simulink model "QBot2_Image_Proc_Line_Following_edited"  (R2015b)
settings: Solver=ode1  StartTime=0.0  StopTime=inf  FixedStep=0.01  RelTol=1e-3
values from neighbouring files (symbols this model uses):
  x = [0 0 0 0 0 0 0 0 0 0 0 0 ... (23417 elements, 23417x1)]    [plot_data.mat]
undefined symbols (not defined in the file or in its folder): HIL, Kinect, qc_get_step_size
libraries: quarc_library x6
settings Model: SimulationMode=external  ExtModeTrigDuration=1  Creator=drmadill  LastModifiedBy=ale
settings SolverCC: PositivePriorityOrder=on
settings DataIOCC: SaveFormat=Array  SignalLoggingSaveFormat=ModelDataLogs
settings OptimizationCC: ExpressionDepthLimit=2147483647
settings DebuggingCC: UnderspecifiedInitializationDetection=Classic  MergeDetectMultiDrivingBlocksExec=none  SolverPrmCheckMsg=warning  FcnCallInpInsideContextMsg=EnableAllAsWarning  AllowSymbolicDim=on  StateNameClashWarn=warning
settings HardwareCC: ProdBitPerPointer=32  ProdLargestAtomicFloat=None  ProdIntDivRoundTo=Undefined  ProdEndianess=Unspecified  ProdWordSize=32  ProdHWDeviceType=32-bit Generic
settings RTWCC: SystemTargetFile=quarc_linux_duovero.tlc  TemplateMakefile=quarc_linux_duovero_tmf  Description=QUARC Linux DuoVero Target
settings STFCustomTargetCC: TargetLibSuffix=.a  TargetPreCompLibLocation=C:\PROGRA~3\QUARC\lib\2015b\LINUX_~1\release  SystemTargetFile=quarc_linux_duovero.tlc
settings GRTTargetCC: TargetLibSuffix=.a  TargetPreCompLibLocation=C:\PROGRA~3\QUARC\lib\2015b\LINUX_~1\release  ParMdlRefBuildCompliant=off  CompOptLevelCompliant=off  GeneratePreprocessorConditionals=Disable all  CombineOutputUpdateFcns=off  MatFileLogging=off  GRTInterface=on  UseToolchainInfoCompliant=off  ExtMode=on  ExtModeMexFile=quarc_comm  ExtModeMexArgs='-w -d /tmp -uri %u', 'tcpip://192.168.2.51:17001'
settings ConfigComp: CovModelRefEnable=Off

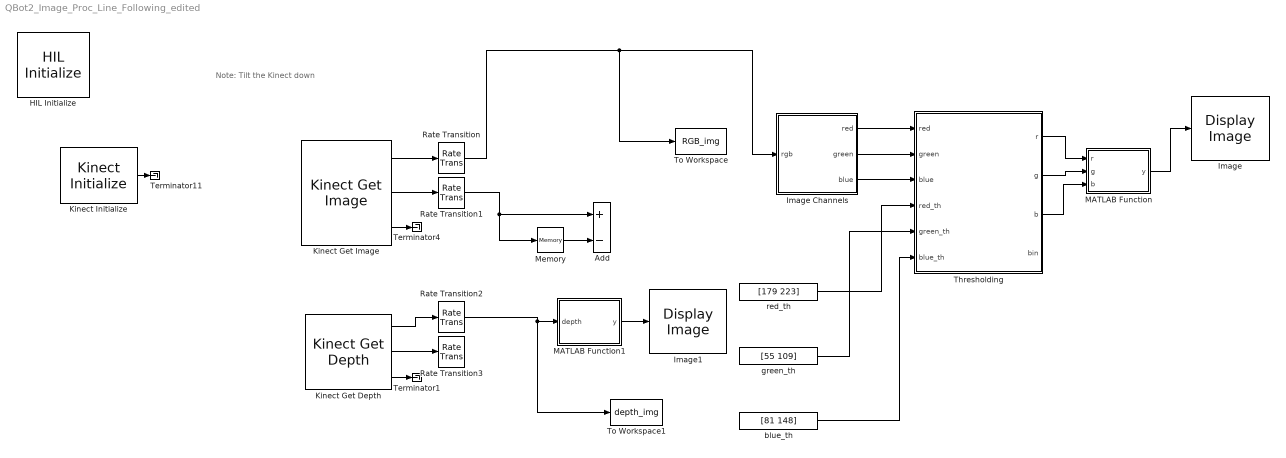
== system QBot2_Image_Proc_Line_Following_edited ==
  note: Note: Tilt the Kinect down
  Add : Sum  Inputs=+-
  HIL Initialize : quarc_library/Data Acquisition/Generic/Configuration/HIL Initialize  Priority=-99  object_name=HIL-1  board_type=qbot2  board_number=0  board_options=enc0_dir=0;enc0_filter=1;enc0_a=0;enc0_b=0;enc0_z=1;enc0_reload=0;enc1_dir=0;enc1_filter=1;enc1_a=0;enc1_b=0;enc1_z=1;enc1_reload=0;pwm0_immediate=0;pwm1_immediate=0;pwm2_immediate=0;pwm3_immediate=0;  exclusive=off  active=off  hardware_clocks=[]  clock_modes=[]  initial_clock_frequencies=[]  set_clock_params_at_start=off  set_clock_params_at_switch_in=off  set_clock_frequencies_at_start=off  set_clock_frequencies_at_switch_in=off  analog_input_channels=[0:9]  analog_input_maximums=[5 5 5 5 16.5 3.3 3.3 3.3 3.3]  analog_input_minimums=[0 0 0 0 0 0 0 0 0]  set_analog_input_params_at_start=off  set_analog_input_params_at_switch_in=off  analog_output_channels=[]  analog_output_maximums=[]  analog_output_minimums=[]  initial_analog_outputs=[]  final_analog_outputs=[]  watchdog_analog_outputs=[]  set_analog_output_params_at_start=off  set_analog_output_params_at_switch_in=off  set_analog_outputs_at_start=off  set_analog_outputs_at_switch_in=off  set_analog_outputs_at_terminate=off  set_analog_outputs_at_switch_out=off  set_analog_outputs_on_watchdog=off  digital_input_channels=[]  digital_output_channels=[]  digital_output_configuration=[]  initial_digital_outputs=[0]  final_digital_outputs=[0]  watchdog_digital_outputs=[0]  set_digital_output_params_at_start=off  set_digital_output_params_at_switch_in=off  set_digital_outputs_at_start=on  set_digital_outputs_at_switch_in=off  set_digital_outputs_at_terminate=on  set_digital_outputs_at_switch_out=off  set_digital_outputs_on_watchdog=on  encoder_channels=[0:3]  quadrature=[4]  encoder_filter_frequency=[]  initial_encoder_counts=[0]  set_encoder_params_at_start=on  set_encoder_params_at_switch_in=off  set_encoder_counts_at_start=on  set_encoder_counts_at_switch_in=off  pwm_channels=[0:3]  pwm_modes=[0]  pwm_frequency=[20e6/1024]  pwm_configuration=[0]  pwm_alignment=[0]  pwm_polarity=[1]  pwm_leading_deadband=[0]  pwm_trailing_deadband=[0]  initial_pwm_outputs=[0]  final_pwm_outputs=[0]  watchdog_pwm_outputs=[0]  set_pwm_params_at_start=on  set_pwm_params_at_switch_in=off  set_pwm_outputs_at_start=on  set_pwm_outputs_at_switch_in=off  set_pwm_outputs_at_terminate=on  set_pwm_outputs_at_switch_out=off  set_pwm_outputs_on_watchdog=on  other_output_channels=[2000:2001 14000 16000]  initial_other_outputs=[0 0 0 7]  final_other_outputs=[0 0 0 7]  watchdog_other_outputs=[]  set_other_outputs_at_start=on  set_other_outputs_at_switch_in=off  set_other_outputs_at_terminate=on  set_other_outputs_at_switch_out=off  set_other_outputs_on_watchdog=off
  Image : quarc_library/Sinks/Figures/Display Image  figure_mode=Use figure window  figure_tag=figure1  axes_tag=axes1  update_rate=1  initial_position="129  195  789  624"  initial_visibility=off  sample_time=-1  axes_only=off  orig_size=off
  Image Channels : Subsystem
  Image1 : quarc_library/Sinks/Figures/Display Image  figure_mode=Use figure window  figure_tag=figure1  axes_tag=axes1  update_rate=1  initial_position="480  173  789  624"  initial_visibility=off  sample_time=-1  axes_only=off  orig_size=off
  Kinect Get Depth : quarc_library/Multimedia/Kinect Get Depth  object_name=Kinect-1  resolution=640 x 480  sample_time=qc_get_step_size * ceil(0.033 / qc_get_step_size)  show_player=off
  Kinect Get Image : quarc_library/Multimedia/Kinect Get Image  object_name=Kinect-1  sensor_type=color  resolution=640 x 480  output_format=MATLAB RGB (HxWx3)  data_type=uint8  backlight=average brightness  flicker=none  brightness=0.2156  gain=1.0  gamma=2.2  autoexposure=on  exposure=0  contrast=1.0  sharpness=0.5  hue=0.0  saturation=1.0  autobalance=on  balance=2700  frame_interval=0  sample_time=qc_get_step_size*10
  Kinect Initialize : quarc_library/Multimedia/Kinect Initialize  object_name=Kinect-1  kinect_type=Kinect for XBox 360  identifier=0  sample_time=qc_get_step_size * 10  active=on
  MATLAB Function : MATLAB Function  TreatAsAtomicUnit=on
  MATLAB Function1 : MATLAB Function  TreatAsAtomicUnit=on
  Memory : Memory
  Rate Transition{,1..3} (4 alike) : RateTransition
  Terminator1 : Terminator
  Terminator11 : Terminator
  Terminator4 : Terminator
  Thresholding : MATLAB Function  TreatAsAtomicUnit=on
  To Workspace : ToWorkspace  VariableName=RGB_img  SampleTime=-1
      settings: MaxDataPoints=1
  To Workspace1 : ToWorkspace  VariableName=depth_img  SampleTime=-1
      settings: MaxDataPoints=1
  blue_th : Constant  Value=[81 148]
  green_th : Constant  Value=[55 109]
  red_th : Constant  Value=[179 223]
  wires:
  Kinect Get Image/1 -> Rate Transition/1
  Kinect Get Image/2 -> Rate Transition1/1
  Rate Transition1/1 -> Memory/1, Add/1
  Memory/1 -> Add/2
  Kinect Get Image/3 -> Terminator4/1
  Rate Transition/1 -> Image Channels/1(rgb), To Workspace/1
  Kinect Initialize/1 -> Terminator11/1
  Kinect Get Depth/1 -> Rate Transition2/1
  Kinect Get Depth/2 -> Rate Transition3/1
  Kinect Get Depth/3 -> Terminator1/1
  Image Channels/2(green) -> Thresholding/2(green)
  Image Channels/1(red) -> Thresholding/1(red)
  Image Channels/3(blue) -> Thresholding/3(blue)
  red_th/1 -> Thresholding/4(red_th)
  green_th/1 -> Thresholding/5(green_th)
  blue_th/1 -> Thresholding/6(blue_th)
  Thresholding/1(r) -> MATLAB Function/1(r)
  Thresholding/2(g) -> MATLAB Function/2(g)
  Thresholding/3(b) -> MATLAB Function/3(b)
  MATLAB Function/1(y) -> Image/1
  Rate Transition2/1 -> MATLAB Function1/1(depth), To Workspace1/1
  MATLAB Function1/1(y) -> Image1/1

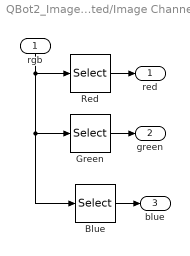
== system QBot2_Image_Proc_Line_Following_edited/Image Channels ==
  rgb : Inport
  Blue : Selector  NumberOfDimensions=3  InputPortWidth=3  IndexOptions=Select all,Select all,Index vector (dialog)  Indices=1,1,3  OutputSizes=1,1,1
  Green : Selector  NumberOfDimensions=3  InputPortWidth=3  IndexOptions=Select all,Select all,Index vector (dialog)  Indices=1,1,2  OutputSizes=1,1,1
  Red : Selector  NumberOfDimensions=3  InputPortWidth=3  IndexOptions=Select all,Select all,Index vector (dialog)  Indices=[1 3],1,1  OutputSizes=1,1,1
  red : Outport
  green : Outport  Port=2
  blue : Outport  Port=3
  wires:
  rgb/1 -> Red/1, Blue/1, Green/1
  Red/1 -> red/1
  Green/1 -> green/1
  Blue/1 -> blue/1

== matlab function QBot2_Image_Proc_Line_Following_edited/MATLAB Function1 ==
  data: depth input; y output
function y = fcn(depth)
%#codegen

y = zeros(size(depth,1), size(depth,2), 3, 'uint8');
y(:,:,1) = uint8(bitand(depth(:,:), 255));
y(:,:,2) = uint8(bitshift(depth(:,:), -4));
y(:,:,3) = uint8(bitshift(depth(:,:), -8));

== matlab function QBot2_Image_Proc_Line_Following_edited/MATLAB Function ==
  data: r input; y output; g input; b input
function y = fcn(r,g,b)
%#codegen

y = zeros(size(r,1), size(r,2), 3, 'uint8');
y(:,:,1) = uint8(r);
y(:,:,2) = uint8(g);
y(:,:,3) = uint8(b);

== matlab function QBot2_Image_Proc_Line_Following_edited/Thresholding ==
  data: red input; r output; g output; b output; bin output; green input; blue input; red_th input; green_th input; blue_th input
function [r, g, b, bin]  = clr_thr(red, ...
    green, blue, red_th, green_th, blue_th)
% This block supports the Embedded MATLAB subset.
% See the help menu for details. 

red_vec = thresh(red, red_th, 1);

green_vec = thresh(green, green_th, 1);

blue_vec = thresh(blue, blue_th, 1);

tmp = double(and(red_vec, green_vec));
tmp_blob = uint8(and(tmp, blue_vec));
bin = uint8(255*tmp_blob);

% background = uint8(255*double(not(tmp_blob)));
% r = uint8(red.*tmp_blob + background);
% g = uint8(green.*tmp_blob + background);
% b = uint8(blue.*tmp_blob + background);

r = uint8(red.*tmp_blob);
g = uint8(green.*tmp_blob);
b = uint8(blue.*tmp_blob);


return;

%--------------------------------------------------------------------------

function x = thresh(x, th, val)

[row col] = size(x);
for i=1:row
    for j=1:col
        if x(i,j) >= th(1) && x(i, j) <= th(2)
            x(i, j) = val;
        else
            x(i, j) = 0;
        end
    end
end

return;

%--------------------------------------------------------------------------
